simulink model "UAV_Research_Environment"  (R2025a)
settings: Solver=ode23t  StartTime=0.0  StopTime=130  MaxStep=2e-3  RelTol=1e-4  AbsTol=1e-3  EnableMultiTasking=on
InitFcn:
  | skipInitialization = false;
  | 
  | if evalin('base', ...
  |         'exist(''CONTROLLER_TUNING_ACTIVE'',''var'')')
  | 
  |     skipInitialization = evalin('base', ...
  |         'logical(CONTROLLER_TUNING_ACTIVE)');
  | end
  | 
  | if ~skipInitialization
  | 
  |     icraControllerPrepared = false;
  | 
  |     hasICRAVariables = evalin('base', ...
  |         ['exist(''AUTOPILOT'',''var'') && ' ...
  |          'exist(''ICRA_ACTIVE_CONTROLLER'',''var'') && ' ...
  |          'exist(''ICRA_ACTIVE_RUN_ID'',''var'')']);
  | 
  |     if hasICRAVariables
  | 
  |         icraControllerPrepared = evalin('base', ...
  |             ['isstruct(AUTOPILOT) && ' ...
  |              'isfield(AUTOPILOT,''info'') && ' ...
  |              'isfield(AUTOPILOT.info,''ICRAControllerID'') && ' ...
  |              'strcmp(string(AUTOPILOT.info.ICRAControllerID), ' ...
  |                     'string(ICRA_ACTIVE_CONTROLLER))']);
  | 
  |     end
  | 
  |     if icraControllerPrepared
  |         skipInitialization = true;
  |     end
  | end
  | 
  | if ~skipInitialization
  | 
  |     mdl = bdroot;
  | 
  |     mdl_file = get_param(mdl, 'FileName');
  | 
  |     project_root = fileparts(mdl_file);
  | 
  |     init_file = fullfile(project_root, 'initialize_project.m');
  | 
  |     if exist(init_file, 'file')
  | 
  |         run(init_file);
  | 
  |     else
  | 
  |         error('initialize_project.m was not found in the model folder.');
  | 
  |     end
  | end
values from neighbouring files (symbols this model uses):
  A_UAV = struct()    [UAV_analytical.m]
  AUTOPILOT = struct()    [UAV_autopilot.m]
  B_UAV = struct()    [UAV_block.m]
  D = A_UAV.source.propeller_diameter_m    [UAV_analytical.m]    (also in plot_controller_results.m = permute(                  D,                  order); plot_estimator_results.m = permute(              D,              order); plot_mission_results.m = permute(                  D,                  order); plot_touchdown_diagnostics.m = permute(                  D,                  order))
  OPERATOR_MODE = OPERATOR_MODE_MANUAL    [initialize_project.m]    (also in uav_remote_gui.m = uint8(0))
  P_ENV = struct()    [Environment.m]
  P_UAV = struct()    [UAV_simscape.m]
  s = sin(angle)    [uav_remote_gui.m]
  SENSOR = struct()    [UAV_sensors.m]
  TRAJECTORY_CONFIG = struct()    [UAV_trajectories.m]
  TRAJECTORY_ID = uint8(          trajectoryIDNumeric)    [UAV_trajectories.m]
  X = reshape(                  D,                  nt,                  [])    [plot_controller_results.m]    (also in plot_estimator_results.m = reshape(              D,              nt,              []); plot_mission_results.m; plot_touchdown_diagnostics.m; plot_trajectory_3d.m)
  Y = absolutePlanNED(1,:)    [plot_trajectory_3d.m]    (also in uav_remote_gui.m = positionNED(:,1))
  Z = landedCGDown -          absolutePlanNED(3,:)    [plot_trajectory_3d.m]    (also in uav_remote_gui.m = landedCGDown-positionNED(:,3))
undefined symbols (not defined in the file or in its folder): Acceleration_ref, F, fractalcoef, Light, MIL, Position_ref, Velocity_ref, Yaw_ref, YawRate_ref
libraries: sm_lib x49, nesl_utility x29, fl_lib x17, slpidlib x16, simulink x14, ee_lib x5, sdl_lib x4, aerolibwind2 x3, aerolibatmos2 x2, sensorbarometerlib x1, sensorgpslib x1, mspsensorlib x1
(part 8 of 9)

== matlab function UAV_Research_Environment/Control Ground Station/Mission Manager/Mission_Manager ==
  settings: updateMethod=DISCRETE
  data: t input; TargetPosition output; RunTrajectoryRequestID input; Position input; Velocity input; MissionPlan input; NumWaypoints input; TargetYaw output; TargetID output; Phase output; Active output; Complete output; NavValid input; MissionDebug output; PassThroughIntermediate input
function [TargetPosition, TargetYaw, TargetID, ...
          Phase, Active, Complete, MissionDebug] = ...
    Mission_Manager( ...
        t, ...
        RunTrajectoryRequestID, ...
        Position, ...
        Velocity, ...
        MissionPlan, ...
        NumWaypoints, ...
        NavValid, ...
        PassThroughIntermediate)

STATUS_WAITING = ...
    uint8(0);

STATUS_ACTIVE = ...
    uint8(1);

STATUS_COMPLETE = ...
    uint8(2);

STATUS_ABORTED = ...
    uint8(3);

persistent lastRunRequestID
persistent missionStatus
persistent currentTargetIndex
persistent activeMissionNumWaypoints
persistent targetCommandID
persistent inHold
persistent holdStartTime

if isempty(lastRunRequestID)

    lastRunRequestID = ...
        uint32(0);

    missionStatus = ...
        STATUS_WAITING;

    currentTargetIndex = ...
        uint16(1);

    activeMissionNumWaypoints = ...
        uint16(0);

    targetCommandID = ...
        uint32(0);

    inHold = ...
        false;

    holdStartTime = ...
        0.0;

end

requestID = ...
    uint32( ...
        RunTrajectoryRequestID);

navigationValid = ...
    logical( ...
        NavValid);

passThroughIntermediate = ...
    logical( ...
        PassThroughIntermediate(1));

numWaypointsRaw = ...
    double( ...
        NumWaypoints);

maxWaypoints = ...
    size( ...
        MissionPlan, ...
        2);

timeValid = ...
    isscalar(t) && ...
    isfinite(t);

positionValid = ...
    numel(Position) >= 3 && ...
    isfinite(Position(1)) && ...
    isfinite(Position(2)) && ...
    isfinite(Position(3));

velocityValid = ...
    numel(Velocity) >= 3 && ...
    isfinite(Velocity(1)) && ...
    isfinite(Velocity(2)) && ...
    isfinite(Velocity(3));

navigationDataValid = ...
    navigationValid && ...
    positionValid && ...
    velocityValid && ...
    timeValid;

numWaypointsValid = ...
    isscalar(numWaypointsRaw) && ...
    isfinite(numWaypointsRaw) && ...
    numWaypointsRaw >= 3 && ...
    numWaypointsRaw <= maxWaypoints && ...
    abs( ...
        numWaypointsRaw - ...
        round(numWaypointsRaw)) < 1e-12;

if numWaypointsValid

    validatedNumWaypoints = ...
        uint16( ...
            round( ...
                numWaypointsRaw));

else

    validatedNumWaypoints = ...
        uint16(0);

end

missionPlanValid = ...
    numWaypointsValid && ...
    size(MissionPlan,1) == 4;

if missionPlanValid

    for columnIndex = 1:maxWaypoints

        if columnIndex <= double(validatedNumWaypoints)

            for rowIndex = 1:4

                if ~isfinite( ...
                        MissionPlan( ...
                            rowIndex, ...
                            columnIndex))

                    missionPlanValid = ...
                        false;

                end

            end

        end

    end

end

homeTargetValid = ...
    size(MissionPlan,1) == 4 && ...
    maxWaypoints >= 1 && ...
    isfinite(MissionPlan(1,1)) && ...
    isfinite(MissionPlan(2,1)) && ...
    isfinite(MissionPlan(3,1)) && ...
    isfinite(MissionPlan(4,1));

if homeTargetValid

    P_HOME = ...
        [ ...
            MissionPlan(1,1);
            MissionPlan(2,1);
            MissionPlan(3,1)
        ];

    Y_HOME = ...
        MissionPlan(4,1);

else

    P_HOME = ...
        zeros(3,1);

    Y_HOME = ...
        0.0;

end

waypointHorizontalTolerance_m = ...
    0.60;

waypointVerticalTolerance_m = ...
    0.20;

waypointSpeedTolerance_m_s = ...
    0.30;

preLandHorizontalTolerance_m = ...
    0.30;

preLandVerticalTolerance_m = ...
    0.15;

preLandSpeedTolerance_m_s = ...
    0.20;

verticalLandingGeometryTolerance_m = ...
    1.0e-6;

waypointHoldTime_s = ...
    0.1;

missionCurrentlyActive = ...
    missionStatus == STATUS_ACTIVE;

numWaypointsChangedDuringMission = ...
    false;

if missionCurrentlyActive

    if numWaypointsValid

        numWaypointsChangedDuringMission = ...
            validatedNumWaypoints ~= ...
            activeMissionNumWaypoints;

    else

        numWaypointsChangedDuringMission = ...
            true;

    end

end

if missionCurrentlyActive && ...
        ( ...
            ~navigationDataValid || ...
            ~missionPlanValid || ...
            numWaypointsChangedDuringMission ...
        )

    missionStatus = ...
        STATUS_ABORTED;

    lastRunRequestID = ...
        requestID;

    inHold = ...
        false;

    if timeValid

        holdStartTime = ...
            t;

    else

        holdStartTime = ...
            0.0;

    end

end

canStartMission = ...
    missionStatus == STATUS_WAITING || ...
    missionStatus == STATUS_COMPLETE || ...
    missionStatus == STATUS_ABORTED;

newMissionRequest = ...
    requestID > uint32(0) && ...
    requestID ~= lastRunRequestID;

if navigationDataValid && ...
        missionPlanValid && ...
        newMissionRequest && ...
        canStartMission

    lastRunRequestID = ...
        requestID;

    missionStatus = ...
        STATUS_ACTIVE;

    activeMissionNumWaypoints = ...
        validatedNumWaypoints;

    currentTargetIndex = ...
        uint16(2);

    inHold = ...
        false;

    targetCommandID = ...
        targetCommandID + ...
        uint32(1);

    holdStartTime = ...
        t;

end

safeTargetIndex = ...
    uint16(1);

if missionStatus == STATUS_ACTIVE

    if activeMissionNumWaypoints >= uint16(3) && ...
            currentTargetIndex >= uint16(2) && ...
            currentTargetIndex <= activeMissionNumWaypoints

        safeTargetIndex = ...
            currentTargetIndex;

    end

elseif missionStatus == STATUS_COMPLETE

    if activeMissionNumWaypoints >= uint16(3)

        safeTargetIndex = ...
            activeMissionNumWaypoints;

    end

end

TargetPosition = ...
    P_HOME;

TargetYaw = ...
    Y_HOME;

Active = ...
    false;

Complete = ...
    false;

if missionStatus == STATUS_ACTIVE && ...
        missionPlanValid

    targetColumn = ...
        double( ...
            safeTargetIndex);

    TargetPosition = ...
        [ ...
            MissionPlan(1,targetColumn);
            MissionPlan(2,targetColumn);
            MissionPlan(3,targetColumn)
        ];

    TargetYaw = ...
        MissionPlan(4,targetColumn);

    Active = ...
        true;

elseif missionStatus == STATUS_COMPLETE && ...
        missionPlanValid

    targetColumn = ...
        double( ...
            safeTargetIndex);

    TargetPosition = ...
        [ ...
            MissionPlan(1,targetColumn);
            MissionPlan(2,targetColumn);
            MissionPlan(3,targetColumn)
        ];

    TargetYaw = ...
        MissionPlan(4,targetColumn);

    Complete = ...
        true;

elseif missionStatus == STATUS_ABORTED

    if positionValid

        TargetPosition = ...
            [ ...
                Position(1);
                Position(2);
                Position(3)
            ];

    else

        TargetPosition = ...
            P_HOME;

    end

    TargetYaw = ...
        Y_HOME;

end

if positionValid

    northError = ...
        Position(1) - ...
        TargetPosition(1);

    eastError = ...
        Position(2) - ...
        TargetPosition(2);

    downError = ...
        Position(3) - ...
        TargetPosition(3);

    horizontalError = ...
        sqrt( ...
            northError*northError + ...
            eastError*eastError);

    verticalError = ...
        abs( ...
            downError);

else

    horizontalError = ...
        inf;

    verticalError = ...
        inf;

end

if velocityValid

    speedMagnitude = ...
        sqrt( ...
            Velocity(1)*Velocity(1) + ...
            Velocity(2)*Velocity(2) + ...
            Velocity(3)*Velocity(3));

else

    speedMagnitude = ...
        inf;

end

preLandAlignmentActive = ...
    false;

if missionStatus == STATUS_ACTIVE && ...
        missionPlanValid && ...
        activeMissionNumWaypoints >= uint16(3)

    currentIndexDouble = ...
        double( ...
            currentTargetIndex);

    finalIndexDouble = ...
        double( ...
            activeMissionNumWaypoints);

    if currentIndexDouble == ...
            finalIndexDouble - 1

        finalSegmentNorth = ...
            MissionPlan(1,finalIndexDouble) - ...
            MissionPlan(1,currentIndexDouble);

        finalSegmentEast = ...
            MissionPlan(2,finalIndexDouble) - ...
            MissionPlan(2,currentIndexDouble);

        finalSegmentHorizontalLength = ...
            sqrt( ...
                finalSegmentNorth*finalSegmentNorth + ...
                finalSegmentEast*finalSegmentEast);

        preLandAlignmentActive = ...
            finalSegmentHorizontalLength <= ...
            verticalLandingGeometryTolerance_m;

    end

end

passThroughActive = ...
    false;

if missionStatus == STATUS_ACTIVE && ...
        passThroughIntermediate && ...
        activeMissionNumWaypoints >= uint16(5)

    currentIndexDouble = ...
        double( ...
            currentTargetIndex);

    finalIndexDouble = ...
        double( ...
            activeMissionNumWaypoints);

    passThroughActive = ...
        currentIndexDouble >= 3 && ...
        currentIndexDouble <= ...
            (finalIndexDouble - 2);

end

if preLandAlignmentActive

    activeHorizontalTolerance_m = ...
        preLandHorizontalTolerance_m;

    activeVerticalTolerance_m = ...
        preLandVerticalTolerance_m;

    activeSpeedTolerance_m_s = ...
        preLandSpeedTolerance_m_s;

else

    activeHorizontalTolerance_m = ...
        waypointHorizontalTolerance_m;

    activeVerticalTolerance_m = ...
        waypointVerticalTolerance_m;

    activeSpeedTolerance_m_s = ...
        waypointSpeedTolerance_m_s;

end

positionOK = ...
    missionStatus == STATUS_ACTIVE && ...
    navigationDataValid && ...
    missionPlanValid && ...
    horizontalError <= activeHorizontalTolerance_m && ...
    verticalError <= activeVerticalTolerance_m;

speedOK = ...
    missionStatus == STATUS_ACTIVE && ...
    navigationDataValid && ...
    missionPlanValid && ...
    speedMagnitude <= activeSpeedTolerance_m_s;

if passThroughActive

    targetReached = ...
        positionOK;

else

    targetReached = ...
        positionOK && ...
        speedOK;

end

if missionStatus == STATUS_ACTIVE && ...
        inHold && ...
        timeValid

    holdElapsedTime = ...
        max( ...
            0.0, ...
            t - holdStartTime);

else

    holdElapsedTime = ...
        0.0;

end

if missionStatus == STATUS_ACTIVE

    currentIndexDouble = ...
        double( ...
            currentTargetIndex);

    finalIndexDouble = ...
        double( ...
            activeMissionNumWaypoints);

    if currentIndexDouble < finalIndexDouble

        if passThroughActive

            if targetReached

                currentTargetIndex = ...
                    currentTargetIndex + ...
                    uint16(1);

                inHold = ...
                    false;

                targetCommandID = ...
                    targetCommandID + ...
                    uint32(1);

                holdStartTime = ...
                    t;

            end

        else

            if ~inHold

                if targetReached

                    inHold = ...
                        true;

                    holdStartTime = ...
                        t;

                end

            else

                if targetReached

                    if (t - holdStartTime) >= ...
                            waypointHoldTime_s

                        currentTargetIndex = ...
                            currentTargetIndex + ...
                            uint16(1);

                        inHold = ...
                            false;

                        targetCommandID = ...
                            targetCommandID + ...
                            uint32(1);

                        holdStartTime = ...
                            t;

                    end

                else

                    holdStartTime = ...
                        t;

                end

            end

        end

    else

        if targetReached

            missionStatus = ...
                STATUS_COMPLETE;

            inHold = ...
                false;

            holdStartTime = ...
                t;

        end

    end

end

TargetPosition = ...
    P_HOME;

TargetYaw = ...
    Y_HOME;

Active = ...
    false;

Complete = ...
    false;

if missionStatus == STATUS_ACTIVE && ...
        missionPlanValid

    targetColumn = ...
        double( ...
            currentTargetIndex);

    if targetColumn >= 2 && ...
            targetColumn <= double(activeMissionNumWaypoints)

        TargetPosition = ...
            [ ...
                MissionPlan(1,targetColumn);
                MissionPlan(2,targetColumn);
                MissionPlan(3,targetColumn)
            ];

        TargetYaw = ...
            MissionPlan(4,targetColumn);

        Active = ...
            true;

    end

elseif missionStatus == STATUS_COMPLETE && ...
        missionPlanValid

    targetColumn = ...
        double( ...
            activeMissionNumWaypoints);

    if targetColumn >= 1 && ...
            targetColumn <= maxWaypoints

        TargetPosition = ...
            [ ...
                MissionPlan(1,targetColumn);
                MissionPlan(2,targetColumn);
                MissionPlan(3,targetColumn)
            ];

        TargetYaw = ...
            MissionPlan(4,targetColumn);

    end

    Complete = ...
        true;

elseif missionStatus == STATUS_ABORTED

    if positionValid

        TargetPosition = ...
            [ ...
                Position(1);
                Position(2);
                Position(3)
            ];

    else

        TargetPosition = ...
            P_HOME;

    end

    TargetYaw = ...
        Y_HOME;

end

if missionStatus == STATUS_WAITING

    phaseValue = ...
        uint16(0);

elseif missionStatus == STATUS_ACTIVE

    targetIndexForPhase = ...
        double( ...
            currentTargetIndex);

    finalIndexForPhase = ...
        double( ...
            activeMissionNumWaypoints);

    if targetIndexForPhase < finalIndexForPhase

        phaseBase = ...
            uint16( ...
                2*targetIndexForPhase - 3);

        if inHold

            phaseValue = ...
                phaseBase + ...
                uint16(1);

        else

            phaseValue = ...
                phaseBase;

        end

    else

        phaseValue = ...
            uint16( ...
                2*finalIndexForPhase - 3);

    end

elseif missionStatus == STATUS_COMPLETE

    phaseValue = ...
        uint16( ...
            2*double(activeMissionNumWaypoints) - 2);

else

    if activeMissionNumWaypoints >= uint16(3)

        phaseNumWaypoints = ...
            double( ...
                activeMissionNumWaypoints);

    elseif validatedNumWaypoints >= uint16(3)

        phaseNumWaypoints = ...
            double( ...
                validatedNumWaypoints);

    else

        phaseNumWaypoints = ...
            3.0;

    end

    phaseValue = ...
        uint16( ...
            2*phaseNumWaypoints - 1);

end

TargetID = ...
    uint32( ...
        targetCommandID);

Phase = ...
    double( ...
        phaseValue);

MissionDebug = ...
    zeros(7,1);

MissionDebug(1) = ...
    horizontalError;

MissionDebug(2) = ...
    verticalError;

MissionDebug(3) = ...
    speedMagnitude;

MissionDebug(4) = ...
    double( ...
        positionOK);

MissionDebug(5) = ...
    double( ...
        speedOK);

MissionDebug(6) = ...
    holdElapsedTime;

MissionDebug(7) = ...
    double( ...
        targetReached);

end

== matlab function UAV_Research_Environment/Control Ground Station/Waypoint Navigator/Waypoint_Navigator ==
  settings: updateMethod=DISCRETE
  data: t input; Position_ref output; MissionPlan input; TargetPosition input; TargetYaw input; TargetID input; Velocity_ref output; Acceleration_ref output; Yaw_ref output; YawRate_ref output; Phase input; Landed input; NumWaypoints input
function [Position_ref, Velocity_ref, Acceleration_ref, ...
          Yaw_ref, YawRate_ref] = ...
    Waypoint_Navigator( ...
        t, ...
        MissionPlan, ...
        TargetPosition, ...
        TargetYaw, ...
        TargetID, ...
        Phase, ...
        Landed, ...
        NumWaypoints)

persistent lastTargetID
persistent lastPhase
persistent segmentStartTime
persistent segmentStartPosition
persistent segmentTargetPosition
persistent segmentDuration
persistent segmentStartYaw
persistent segmentTargetYaw
persistent segmentYawDelta
persistent yawMotionDuration
persistent yawStageDuration
persistent segmentIsLanding
persistent referencePosition
persistent referenceYaw
persistent referenceInitialized

if isempty(lastTargetID)

    lastTargetID = ...
        uint32(0);

    lastPhase = ...
        -1.0;

    segmentStartTime = ...
        0.0;

    segmentStartPosition = ...
        zeros(3,1);

    segmentTargetPosition = ...
        zeros(3,1);

    segmentDuration = ...
        1.0;

    segmentStartYaw = ...
        0.0;

    segmentTargetYaw = ...
        0.0;

    segmentYawDelta = ...
        0.0;

    yawMotionDuration = ...
        0.0;

    yawStageDuration = ...
        0.0;

    segmentIsLanding = ...
        false;

    referencePosition = ...
        zeros(3,1);

    referenceYaw = ...
        0.0;

    referenceInitialized = ...
        false;

end

horizontalSpeedMax_m_s = ...
    1.40;

horizontalAccelerationMax_m_s2 = ...
    1.25;

horizontalJerkMax_m_s3 = ...
    2.50;

climbSpeedMax_m_s = ...
    1.10;

descentSpeedMax_m_s = ...
    0.70;

landingDescentSpeedMax_m_s = ...
    0.45;

verticalAccelerationMax_m_s2 = ...
    1.00;

verticalJerkMax_m_s3 = ...
    2.00;

YawRateMax_rad_s = ...
    pi / 3.0;          % 60 deg/s

YawAccelerationMax_rad_s2 = ...
    pi / 2.0;          % 90 deg/s^2

YawJerkMax_rad_s3 = ...
    pi;                % 180 deg/s^3

yawChangeTolerance_rad = ...
    pi / 360.0;

minimumYawMotionTime_s = ...
    0.50;

yawSettlingTime_s = ...
    0.25;

minimumSegmentTime_s = ...
    0.50;


currentPhase = ...
    round( ...
        double(Phase));

currentTargetID = ...
    uint32( ...
        TargetID);

numWaypointsRaw = ...
    double( ...
        NumWaypoints);

maxWaypoints = ...
    size( ...
        MissionPlan, ...
        2);

numWaypointsValid = ...
    isscalar(numWaypointsRaw) && ...
    isfinite(numWaypointsRaw) && ...
    numWaypointsRaw >= 3 && ...
    numWaypointsRaw <= maxWaypoints && ...
    abs( ...
        numWaypointsRaw - ...
        round(numWaypointsRaw)) < 1.0e-12;

if numWaypointsValid

    activeNumWaypoints = ...
        round( ...
            numWaypointsRaw);

else

    activeNumWaypoints = ...
        0.0;

end

missionPlanValid = ...
    numWaypointsValid && ...
    size(MissionPlan,1) == 4;

if missionPlanValid

    for columnIndex = 1:maxWaypoints

        if columnIndex <= activeNumWaypoints

            for rowIndex = 1:4

                if ~isfinite( ...
                        MissionPlan( ...
                            rowIndex, ...
                            columnIndex))

                    missionPlanValid = ...
                        false;

                end

            end

        end

    end

end


if missionPlanValid

    P_HOME = ...
        [ ...
            MissionPlan(1,1);
            MissionPlan(2,1);
            MissionPlan(3,1)
        ];

    Y_HOME_RAW = ...
        MissionPlan(4,1);

    landColumn = ...
        activeNumWaypoints;

    P_LAND = ...
        [ ...
            MissionPlan(1,landColumn);
            MissionPlan(2,landColumn);
            MissionPlan(3,landColumn)
        ];

    Y_LAND_RAW = ...
        MissionPlan(4,landColumn);

    Y_HOME = ...
        atan2( ...
            sin(Y_HOME_RAW), ...
            cos(Y_HOME_RAW));

    Y_LAND = ...
        atan2( ...
            sin(Y_LAND_RAW), ...
            cos(Y_LAND_RAW));

    landingPhase = ...
        2.0*activeNumWaypoints - ...
        3.0;

else

    P_HOME = ...
        zeros(3,1);

    Y_HOME = ...
        0.0;

    P_LAND = ...
        zeros(3,1);

    Y_LAND = ...
        0.0;

    landingPhase = ...
        inf;

end

timeValid = ...
    isscalar(t) && ...
    isfinite(t);

targetPositionValid = ...
    numel(TargetPosition) >= 3 && ...
    isfinite(TargetPosition(1)) && ...
    isfinite(TargetPosition(2)) && ...
    isfinite(TargetPosition(3));

targetYawValid = ...
    isscalar(TargetYaw) && ...
    isfinite(TargetYaw);


if ~referenceInitialized

    if missionPlanValid

        referencePosition = ...
            P_HOME;

        referenceYaw = ...
            Y_HOME;

        segmentStartPosition = ...
            P_HOME;

        segmentTargetPosition = ...
            P_HOME;

        segmentStartYaw = ...
            Y_HOME;

        segmentTargetYaw = ...
            Y_HOME;

        segmentYawDelta = ...
            0.0;

        if timeValid

            segmentStartTime = ...
                t;

        else

            segmentStartTime = ...
                0.0;

        end

        segmentDuration = ...
            minimumSegmentTime_s;

        yawMotionDuration = ...
            0.0;

        yawStageDuration = ...
            0.0;

        segmentIsLanding = ...
            false;

        referenceInitialized = ...
            true;

    else

        Position_ref = ...
            referencePosition;

        Velocity_ref = ...
            zeros(3,1);

        Acceleration_ref = ...
            zeros(3,1);

        Yaw_ref = ...
            referenceYaw;

        YawRate_ref = ...
            0.0;

        return;

    end

end

if ~missionPlanValid || ...
        ~timeValid || ...
        ~targetPositionValid

    Position_ref = ...
        referencePosition;

    Velocity_ref = ...
        zeros(3,1);

    Acceleration_ref = ...
        zeros(3,1);

    Yaw_ref = ...
        referenceYaw;

    YawRate_ref = ...
        0.0;

    return;

end

if targetYawValid

    effectiveInputTargetYaw = ...
        TargetYaw;

else

    effectiveInputTargetYaw = ...
        referenceYaw;

end


if currentTargetID == uint32(0)

    referencePosition = ...
        P_HOME;

    referenceYaw = ...
        Y_HOME;

    segmentStartPosition = ...
        P_HOME;

    segmentTargetPosition = ...
        P_HOME;

    segmentStartYaw = ...
        Y_HOME;

    segmentTargetYaw = ...
        Y_HOME;

    segmentYawDelta = ...
        0.0;

    yawMotionDuration = ...
        0.0;

    yawStageDuration = ...
        0.0;

    segmentIsLanding = ...
        false;

    Position_ref = ...
        P_HOME;

    Velocity_ref = ...
        zeros(3,1);

    Acceleration_ref = ...
        zeros(3,1);

    Yaw_ref = ...
        Y_HOME;

    YawRate_ref = ...
        0.0;

    lastPhase = ...
        double(currentPhase);

    return;

end


if logical(Landed) && ...
        currentPhase >= landingPhase

    referencePosition = ...
        P_LAND;

    referenceYaw = ...
        Y_LAND;

    segmentStartPosition = ...
        P_LAND;

    segmentTargetPosition = ...
        P_LAND;

    segmentStartYaw = ...
        Y_LAND;

    segmentTargetYaw = ...
        Y_LAND;

    segmentYawDelta = ...
        0.0;

    yawMotionDuration = ...
        0.0;

    yawStageDuration = ...
        0.0;

    segmentIsLanding = ...
        true;

    Position_ref = ...
        P_LAND;

    Velocity_ref = ...
        zeros(3,1);

    Acceleration_ref = ...
        zeros(3,1);

    Yaw_ref = ...
        Y_LAND;

    YawRate_ref = ...
        0.0;

    lastPhase = ...
        double(currentPhase);

    return;

end

enteringLanding = ...
    currentPhase == landingPhase && ...
    round(lastPhase) ~= landingPhase;

newTarget = ...
    currentTargetID ~= lastTargetID;

if newTarget || enteringLanding

    previousTargetID = ...
        lastTargetID;

    lastTargetID = ...
        currentTargetID;

    segmentStartTime = ...
        t;

    if previousTargetID == uint32(0)

        segmentStartPosition = ...
            P_HOME;

        referencePosition = ...
            P_HOME;

        segmentStartYaw = ...
            Y_HOME;

        referenceYaw = ...
            Y_HOME;

    else

        segmentStartPosition = ...
            referencePosition;

        segmentStartYaw = ...
            referenceYaw;

    end

    segmentIsLanding = ...
        currentPhase == landingPhase;

    if segmentIsLanding

        segmentTargetPosition = ...
            P_LAND;

        effectiveTargetYaw = ...
            Y_LAND;

    else

        segmentTargetPosition = ...
            [ ...
                TargetPosition(1);
                TargetPosition(2);
                TargetPosition(3)
            ];

        effectiveTargetYaw = ...
            effectiveInputTargetYaw;

    end

    effectiveTargetYaw = ...
        atan2( ...
            sin(effectiveTargetYaw), ...
            cos(effectiveTargetYaw));

    segmentTargetYaw = ...
        effectiveTargetYaw;

    rawYawDelta = ...
        segmentTargetYaw - ...
        segmentStartYaw;

    segmentYawDelta = ...
        atan2( ...
            sin(rawYawDelta), ...
            cos(rawYawDelta));

    yawDistance = ...
        abs( ...
            segmentYawDelta);

    if yawDistance <= yawChangeTolerance_rad

        segmentYawDelta = ...
            0.0;

        segmentStartYaw = ...
            segmentTargetYaw;

        referenceYaw = ...
            segmentTargetYaw;

        yawMotionDuration = ...
            0.0;

        yawStageDuration = ...
            0.0;

    else

        yawTimeRate = ...
            1.875 * ...
            yawDistance / ...
            YawRateMax_rad_s;

        yawTimeAcceleration = ...
            sqrt( ...
                5.7735026919 * ...
                yawDistance / ...
                YawAccelerationMax_rad_s2);

        yawTimeJerk = ...
            ( ...
                60.0 * ...
                yawDistance / ...
                YawJerkMax_rad_s3 ...
            ) ^ (1.0/3.0);

        yawMotionDuration = ...
            minimumYawMotionTime_s;

        if yawTimeRate > yawMotionDuration

            yawMotionDuration = ...
                yawTimeRate;

        end

        if yawTimeAcceleration > yawMotionDuration

            yawMotionDuration = ...
                yawTimeAcceleration;

        end

        if yawTimeJerk > yawMotionDuration

            yawMotionDuration = ...
                yawTimeJerk;

        end

        if ~isfinite(yawMotionDuration) || ...
                yawMotionDuration < minimumYawMotionTime_s

            yawMotionDuration = ...
                minimumYawMotionTime_s;

        end

        yawStageDuration = ...
            yawMotionDuration + ...
            yawSettlingTime_s;

    end

    deltaPosition = ...
        segmentTargetPosition - ...
        segmentStartPosition;

    horizontalDistance = ...
        sqrt( ...
            deltaPosition(1)*deltaPosition(1) + ...
            deltaPosition(2)*deltaPosition(2));

    verticalDistance = ...
        abs( ...
            deltaPosition(3));

    horizontalTimeSpeed = ...
        0.0;

    horizontalTimeAcceleration = ...
        0.0;

    horizontalTimeJerk = ...
        0.0;

    if horizontalDistance > 0.0

        horizontalTimeSpeed = ...
            1.875 * ...
            horizontalDistance / ...
            horizontalSpeedMax_m_s;

        horizontalTimeAcceleration = ...
            sqrt( ...
                5.7735026919 * ...
                horizontalDistance / ...
                horizontalAccelerationMax_m_s2);

        horizontalTimeJerk = ...
            ( ...
                60.0 * ...
                horizontalDistance / ...
                horizontalJerkMax_m_s3 ...
            ) ^ (1.0/3.0);

    end

    verticalSpeedMax = ...
        descentSpeedMax_m_s;

    if deltaPosition(3) < 0.0

        verticalSpeedMax = ...
            climbSpeedMax_m_s;

    elseif segmentIsLanding

        verticalSpeedMax = ...
            landingDescentSpeedMax_m_s;

    end

    verticalTimeSpeed = ...
        0.0;

    verticalTimeAcceleration = ...
        0.0;

    verticalTimeJerk = ...
        0.0;

    if verticalDistance > 0.0

        verticalTimeSpeed = ...
            1.875 * ...
            verticalDistance / ...
            verticalSpeedMax;

        verticalTimeAcceleration = ...
            sqrt( ...
                5.7735026919 * ...
                verticalDistance / ...
                verticalAccelerationMax_m_s2);

        verticalTimeJerk = ...
            ( ...
                60.0 * ...
                verticalDistance / ...
                verticalJerkMax_m_s3 ...
            ) ^ (1.0/3.0);

    end

    segmentDuration = ...
        minimumSegmentTime_s;

    if horizontalTimeSpeed > segmentDuration

        segmentDuration = ...
            horizontalTimeSpeed;

    end

    if horizontalTimeAcceleration > segmentDuration

        segmentDuration = ...
            horizontalTimeAcceleration;

    end

    if horizontalTimeJerk > segmentDuration

        segmentDuration = ...
            horizontalTimeJerk;

    end

    if verticalTimeSpeed > segmentDuration

        segmentDuration = ...
            verticalTimeSpeed;

    end

    if verticalTimeAcceleration > segmentDuration

        segmentDuration = ...
            verticalTimeAcceleration;

    end

    if verticalTimeJerk > segmentDuration

        segmentDuration = ...
            verticalTimeJerk;

    end

    if yawStageDuration > segmentDuration

        segmentDuration = ...
            yawStageDuration;

    end

    if ~isfinite(segmentDuration) || ...
            segmentDuration < minimumSegmentTime_s

        segmentDuration = ...
            minimumSegmentTime_s;

    end

end

lastPhase = ...
    double(currentPhase);

elapsedTime = ...
    t - ...
    segmentStartTime;

if elapsedTime < 0.0 || ...
        ~isfinite(elapsedTime)

    elapsedTime = ...
        0.0;

end

if elapsedTime >= segmentDuration

    if segmentIsLanding

        Position_ref = ...
            P_LAND;

        segmentTargetPosition = ...
            P_LAND;

    else

        Position_ref = ...
            segmentTargetPosition;

    end

    Velocity_ref = ...
        zeros(3,1);

    Acceleration_ref = ...
        zeros(3,1);

else

    tau = ...
        elapsedTime / ...
        segmentDuration;

    if tau < 0.0

        tau = ...
            0.0;

    elseif tau > 1.0

        tau = ...
            1.0;

    end

    tau2 = ...
        tau*tau;

    tau3 = ...
        tau2*tau;

    tau4 = ...
        tau3*tau;

    tau5 = ...
        tau4*tau;

    s = ...
        10.0*tau3 - ...
        15.0*tau4 + ...
         6.0*tau5;

    sDot = ...
        ( ...
            30.0*tau2 - ...
            60.0*tau3 + ...
            30.0*tau4 ...
        ) / segmentDuration;

    sDDot = ...
        ( ...
            60.0*tau - ...
            180.0*tau2 + ...
            120.0*tau3 ...
        ) / ...
        (segmentDuration*segmentDuration);

    deltaPosition = ...
        segmentTargetPosition - ...
        segmentStartPosition;

    Position_ref = ...
        segmentStartPosition + ...
        s*deltaPosition;

    Velocity_ref = ...
        sDot*deltaPosition;

    Acceleration_ref = ...
        sDDot*deltaPosition;

end

if segmentIsLanding

    landingStartDown = ...
        segmentStartPosition(3);

    landingTargetDown = ...
        P_LAND(3);

    if landingTargetDown >= landingStartDown

        if Position_ref(3) > landingTargetDown

            Position_ref(3) = ...
                landingTargetDown;

            Velocity_ref(3) = ...
                0.0;

            Acceleration_ref(3) = ...
                0.0;

        end

    else

        if Position_ref(3) < landingTargetDown

            Position_ref(3) = ...
                landingTargetDown;

            Velocity_ref(3) = ...
                0.0;

            Acceleration_ref(3) = ...
                0.0;

        end

    end

    if abs( ...
            Position_ref(3) - ...
            landingTargetDown) < 1.0e-10

        Position_ref(3) = ...
            landingTargetDown;

    end

end

if yawMotionDuration > 0.0 && ...
        elapsedTime < yawMotionDuration

    tauYaw = ...
        elapsedTime / ...
        yawMotionDuration;

    if tauYaw < 0.0

        tauYaw = ...
            0.0;

    elseif tauYaw > 1.0

        tauYaw = ...
            1.0;

    end

    tauYaw2 = ...
        tauYaw*tauYaw;

    tauYaw3 = ...
        tauYaw2*tauYaw;

    tauYaw4 = ...
        tauYaw3*tauYaw;

    tauYaw5 = ...
        tauYaw4*tauYaw;

    sYaw = ...
        10.0*tauYaw3 - ...
        15.0*tauYaw4 + ...
         6.0*tauYaw5;

    sYawDot = ...
        ( ...
            30.0*tauYaw2 - ...
            60.0*tauYaw3 + ...
            30.0*tauYaw4 ...
        ) / ...
        yawMotionDuration;

    yawContinuous = ...
        segmentStartYaw + ...
        sYaw*segmentYawDelta;

    Yaw_ref = ...
        atan2( ...
            sin(yawContinuous), ...
            cos(yawContinuous));

    YawRate_ref = ...
        sYawDot * ...
        segmentYawDelta;

else

    yawEndpointContinuous = ...
        segmentStartYaw + ...
        segmentYawDelta;

    Yaw_ref = ...
        atan2( ...
            sin(yawEndpointContinuous), ...
            cos(yawEndpointContinuous));

    YawRate_ref = ...
        0.0;

end

referencePosition = ...
    Position_ref;

referenceYaw = ...
    Yaw_ref;

end

== matlab function UAV_Research_Environment/Autopilot/Motor Command/Motor Spool Logic ==
  data: mode input; u input; y output
function y = Motor_Spool_Logic(mode, u)

Ts = 0.005;
spoolDownTime_s = 1.00;

persistent previousMode
persistent previousOutput
persistent spoolStartOmega
persistent spoolElapsedTime
persistent spoolActive

if isempty(previousMode)

    previousMode = ...
        double(mode);

end

if isempty(previousOutput)

    previousOutput = ...
        double(u);

end

if isempty(spoolStartOmega)

    spoolStartOmega = ...
        double(u);

end

if isempty(spoolElapsedTime)

    spoolElapsedTime = ...
        0.0;

end

if isempty(spoolActive)

    spoolActive = ...
        false;

end

currentMode = ...
    double(mode);

targetOmega = ...
    double(u);

comingFromFlight = ...
    previousMode >= 3 && ...
    previousMode <= 6;

enteringArmedIdle = ...
    currentMode == 2 && ...
    previousMode ~= 2;

if enteringArmedIdle && comingFromFlight

    spoolActive = ...
        true;

    spoolStartOmega = ...
        previousOutput;

    spoolElapsedTime = ...
        0.0;

end

if currentMode == 1

    y = ...
        targetOmega;

    spoolActive = ...
        false;

    spoolElapsedTime = ...
        0.0;

elseif currentMode == 2 && spoolActive

    spoolElapsedTime = ...
        spoolElapsedTime + Ts;

    alpha = ...
        spoolElapsedTime / ...
        spoolDownTime_s;

    alpha = ...
        min( ...
            max(alpha,0.0), ...
            1.0);

    y = ...
        spoolStartOmega + ...
        alpha .* ...
        (targetOmega-spoolStartOmega);

    if alpha >= 1.0

        y = ...
            targetOmega;

        spoolActive = ...
            false;

    end

else

    y = ...
        targetOmega;

    spoolActive = ...
        false;

    spoolElapsedTime = ...
        0.0;

end

previousOutput = ...
    y;

previousMode = ...
    currentMode;

end

== matlab function UAV_Research_Environment/Remote Controller/Automatic Operator/Automatic Protocol ==
  data: t input; ArmCommand output; TrajectoryID input; ProtocolTable_s input; RunTrajectoryRequestID output
function [ArmCommand,RunTrajectoryRequestID] = ...
    Automatic_Protocol(t,TrajectoryID,ProtocolTable_s)
%#codegen

ArmCommand = false;
RunTrajectoryRequestID = uint32(0);

trajectoryIndex = double(TrajectoryID(1)); %#ok<NASGU>

simulationTime_s = double(t(1));

armTime_s = double(ProtocolTable_s(1));
runTime_s = double(ProtocolTable_s(2));
disarmTime_s = double(ProtocolTable_s(3));

if simulationTime_s >= armTime_s && ...
        simulationTime_s < disarmTime_s

    ArmCommand = true;
end

if simulationTime_s >= runTime_s

    RunTrajectoryRequestID = uint32(1);
end

end

== matlab function UAV_Research_Environment/Control Ground Station/Home Manager ==
  settings: updateMethod=DISCRETE
  data: HomePositionSource input; HomePosition output; ArmCommand input; HomeValid output
function [HomePosition, HomeValid] = ...
    Home_Manager( ...
        HomePositionSource, ...
        ArmCommand)

persistent storedHome
persistent storedHomeValid
persistent previousArmCommand

if isempty(previousArmCommand)

    storedHome = ...
        zeros(3,1);

    storedHomeValid = ...
        false;

    previousArmCommand = ...
        false;

end

currentArmCommand = ...
    logical( ...
        ArmCommand);

armRisingEdge = ...
    currentArmCommand && ...
    ~previousArmCommand;

homeSourceValid = ...
    numel(HomePositionSource) == 3 && ...
    all( ...
        isfinite( ...
            HomePositionSource));

if armRisingEdge

    if homeSourceValid

        storedHome = ...
            reshape( ...
                HomePositionSource, ...
                3, ...
                1);

        storedHomeValid = ...
            true;

    else

        storedHomeValid = ...
            false;

    end

end

previousArmCommand = ...
    currentArmCommand;

HomePosition = ...
    storedHome;

HomeValid = ...
    storedHomeValid;

end
